simulink model "Guidance_Equations2"  (R2013a)
settings: Solver=ode4  StartTime=0.0  StopTime=10  FixedStep=0.01  RelTol=1e-3
undefined symbols (not defined in the file or in its folder): sigbuilder_block
settings Model: Creator=Ibrahim_B92  LastModifiedBy=Ibrahim_B92
settings DataIOCC: LimitDataPoints=off  SaveOutput=off

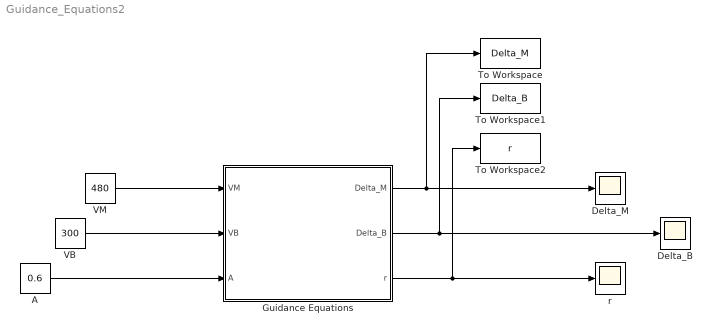
== system Guidance_Equations2 ==
  A : Constant  Value=0.6
  Delta_B : Scope
  Delta_M : Scope
      settings: YMin=0.6683  YMax=0.67
  Guidance Equations : Subsystem
  To Workspace : ToWorkspace  VariableName=Delta_M  SampleTime=-1
  To Workspace1 : ToWorkspace  VariableName=Delta_B  SampleTime=-1
  To Workspace2 : ToWorkspace  VariableName=r  SampleTime=-1
  VB : Constant  Value=300
  VM : Constant  Value=480
  r : Scope
      settings: SaveName=ScopeData2
  wires:
  VM/1 -> Guidance Equations/1(VM)
  VB/1 -> Guidance Equations/2(VB)
  Guidance Equations/1(Delta_M) -> Delta_M/1, To Workspace/1
  Guidance Equations/2(Delta_B) -> Delta_B/1, To Workspace1/1
  Guidance Equations/3(r) -> To Workspace2/1, r/1
  A/1 -> Guidance Equations/3(A)

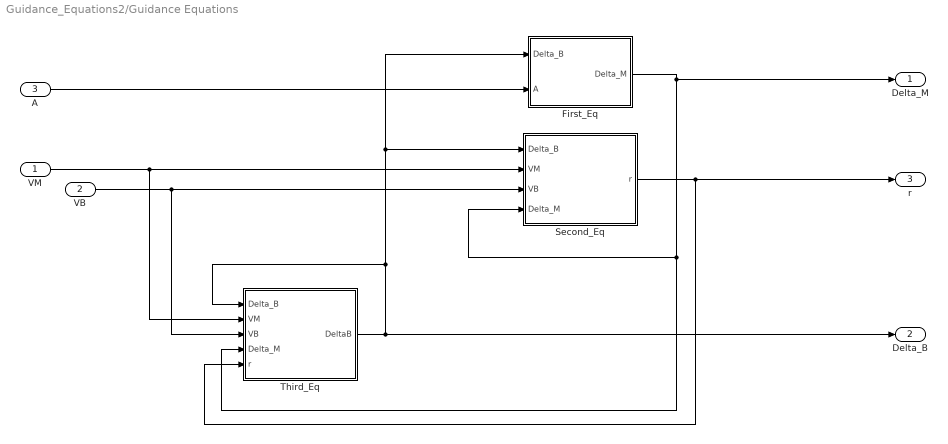
== system Guidance_Equations2/Guidance Equations ==
  VM : Inport
  VB : Inport  Port=2
  A : Inport  Port=3
  First_Eq : Subsystem
  Second_Eq : Subsystem
  Third_Eq : Subsystem
  Delta_M : Outport
  Delta_B : Outport  Port=2
  r : Outport  Port=3
  wires:
  Third_Eq/1(DeltaB) -> Second_Eq/1(Delta_B), First_Eq/1(Delta_B), Third_Eq/1(Delta_B), Delta_B/1
  First_Eq/1(Delta_M) -> Delta_M/1, Third_Eq/4(Delta_M), Second_Eq/4(Delta_M)
  VM/1 -> Third_Eq/2(VM), Second_Eq/2(VM)
  VB/1 -> Third_Eq/3(VB), Second_Eq/3(VB)
  Second_Eq/1(r) -> Third_Eq/5(r), r/1
  A/1 -> First_Eq/2(A)

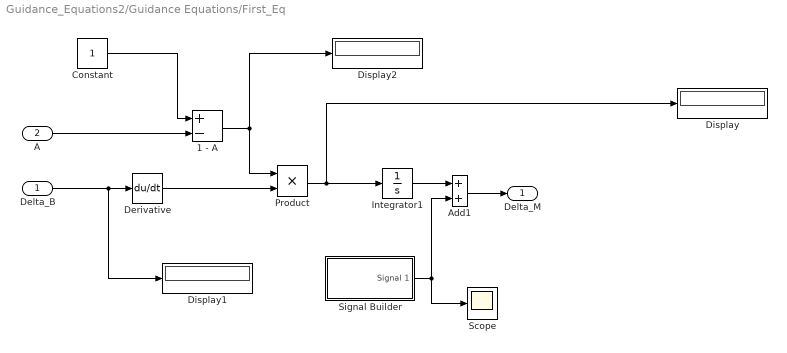
== system Guidance_Equations2/Guidance Equations/First_Eq ==
  Delta_B : Inport
  A : Inport  Port=2
  1 - A : Sum  Inputs=+-
  Add1 : Sum
  Constant : Constant
  Derivative : Derivative
  Display : Display
  Display1 : Display
  Display2 : Display
  Integrator1 : Integrator
  Product : Product
  Scope : Scope
      settings: SaveName=ScopeData4
  Signal Builder : Subsystem  Tag=STV Subsys  LoadFcn=sigbuilder_block('load',[437.25 118.5 550.5 394.5 ]);  StartFcn=sigbuilder_block('start');  StopFcn=sigbuilder_block('stop');  ClipboardFcn=sigbuilder_block('clipboard');  mask(Sigbuilder block){}
      mask help: Simulink:masks:SigbuilderBlock_MD
      mask init:
      | if ~strcmp(get_param(bdroot(gcbh),'SimulationStatus'),'stopped') tuvar = sigbuilder_block('maskInit'); end
      settings: CopyFcn=sigbuilder_block('copy');  DeleteFcn=sigbuilder_block('delete');  ModelCloseFcn=sigbuilder_block('modelClose');  PreSaveFcn=sigbuilder_block('preSave');  PauseFcn=sigbuilder_block('pause');  ContinueFcn=sigbuilder_block('continue');  NameChangeFcn=sigbuilder_block('namechange');  OpenFcn=sigbuilder_block('open',[437.25 118.5 550.5 394.5 ]);  CloseFcn=sigbuilder_block('close');
      mask Display: plot(0, 0, 100, 100,[2, 2, 32, 32, 2], [68, 8, 8, 68, 68],[32, 2], [38, 38], [32, 19, 2],[53, 60, 44], [32, 17, 17, 2],[16, 16, 31, 31]);txt = getActiveGroup(gcbh);text(2, 100, txt,'verticalAlignment', 'top');
  Delta_M : Outport
  wires:
  Delta_B/1 -> Display1/1, Derivative/1
  Derivative/1 -> Product/2
  Product/1 -> Display/1, Integrator1/1
  A/1 -> 1 - A/2
  Constant/1 -> 1 - A/1
  1 - A/1 -> Display2/1, Product/1
  Signal Builder/1(Signal 1) -> Add1/2, Scope/1
  Add1/1 -> Delta_M/1
  Integrator1/1 -> Add1/1

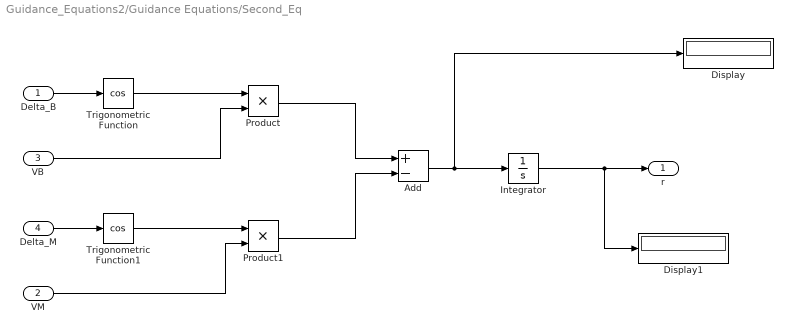
== system Guidance_Equations2/Guidance Equations/Second_Eq ==
  Delta_B : Inport
  VM : Inport  Port=2
  VB : Inport  Port=3
  Delta_M : Inport  Port=4
  Add : Sum  Inputs=+-
  Display : Display
  Display1 : Display
  Integrator : Integrator
  Product : Product
  Product1 : Product
  Trigonometric Function : Trigonometry  Operator=cos
  Trigonometric Function1 : Trigonometry  Operator=cos
  r : Outport
  wires:
  Delta_B/1 -> Trigonometric Function/1
  VB/1 -> Product/2
  VM/1 -> Product1/2
  Product/1 -> Add/1
  Product1/1 -> Add/2
  Add/1 -> Integrator/1, Display/1
  Delta_M/1 -> Trigonometric Function1/1
  Trigonometric Function1/1 -> Product1/1
  Trigonometric Function/1 -> Product/1
  Integrator/1 -> Display1/1, r/1

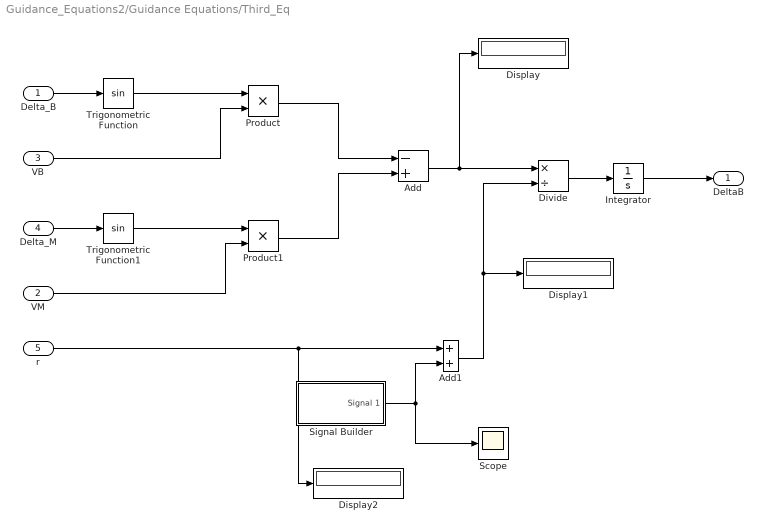
== system Guidance_Equations2/Guidance Equations/Third_Eq ==
  Delta_B : Inport
  VM : Inport  Port=2
  VB : Inport  Port=3
  Delta_M : Inport  Port=4
  r : Inport  Port=5
  Add : Sum  Inputs=-+
  Add1 : Sum
  Display : Display
  Display1 : Display
  Display2 : Display
  Divide : Product  Inputs=*/
  Integrator : Integrator
  Product : Product
  Product1 : Product
  Scope : Scope
      settings: SaveName=ScopeData3
  Signal Builder : Subsystem  Tag=STV Subsys  LoadFcn=sigbuilder_block('load');  StartFcn=sigbuilder_block('start');  StopFcn=sigbuilder_block('stop');  ClipboardFcn=sigbuilder_block('clipboard');  mask(Sigbuilder block){}
      mask help: Simulink:masks:SigbuilderBlock_MD
      mask init:
      | if ~strcmp(get_param(bdroot(gcbh),'SimulationStatus'),'stopped') tuvar = sigbuilder_block('maskInit'); end
      settings: CopyFcn=sigbuilder_block('copy');  DeleteFcn=sigbuilder_block('delete');  ModelCloseFcn=sigbuilder_block('modelClose');  PreSaveFcn=sigbuilder_block('preSave');  PauseFcn=sigbuilder_block('pause');  ContinueFcn=sigbuilder_block('continue');  NameChangeFcn=sigbuilder_block('namechange');  OpenFcn=sigbuilder_block('open',[437.25 118.5 550.5 394.5 ]);  CloseFcn=sigbuilder_block('close');
      mask Display: plot(0, 0, 100, 100,[2, 2, 32, 32, 2], [68, 8, 8, 68, 68],[32, 2], [38, 38], [32, 19, 2],[53, 60, 44], [32, 17, 17, 2],[16, 16, 31, 31]);txt = getActiveGroup(gcbh);text(2, 100, txt,'verticalAlignment', 'top');
  Trigonometric Function : Trigonometry
  Trigonometric Function1 : Trigonometry
  DeltaB : Outport
  wires:
  Delta_B/1 -> Trigonometric Function/1
  Delta_M/1 -> Trigonometric Function1/1
  VB/1 -> Product/2
  VM/1 -> Product1/2
  Integrator/1 -> DeltaB/1
  Add/1 -> Display/1, Divide/1
  Divide/1 -> Integrator/1
  r/1 -> Add1/1, Display2/1
  Trigonometric Function1/1 -> Product1/1
  Product/1 -> Add/1
  Product1/1 -> Add/2
  Trigonometric Function/1 -> Product/1
  Add1/1 -> Display1/1, Divide/2
  Signal Builder/1(Signal 1) -> Add1/2, Scope/1

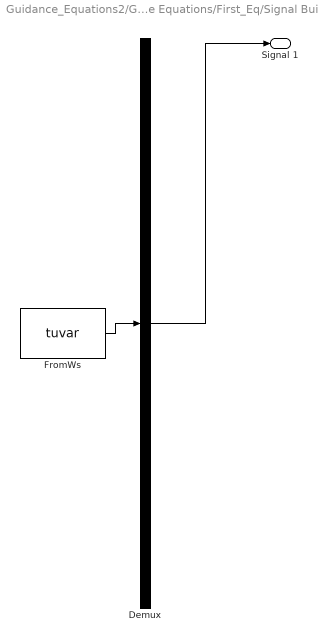
== system Guidance_Equations2/Guidance Equations/First_Eq/Signal Builder ==
  Demux : Demux  Tag=STV Demux  Outputs=1
  FromWs : FromWorkspace  Tag=STV FromWs  VariableName=tuvar  SampleTime=0
      SigBuilderData=|
      | common.afterFinalStr = 'Extrapolate'
      | common.sampleTime = 0
      | dataSet.timeRange = [0 10]
      | dataSet.name = 'Group 1'
      | sbobj.Groups.Name = 'Group 1'
      | sbobj.Groups.Signals.Name = 'Signal 1'
      | sbobj.Groups.Signals.XData = [0 0.01 0.01 10]
      | sbobj.Groups.Signals.YData = [1 1 0 0]
  Signal 1 : Outport  Tag=STV Outport
  wires:
  Demux/1 -> Signal 1/1
  FromWs/1 -> Demux/1

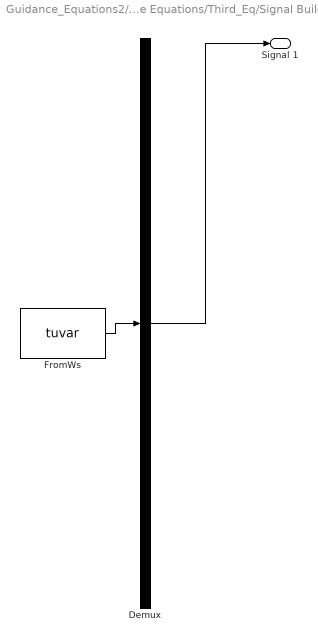
== system Guidance_Equations2/Guidance Equations/Third_Eq/Signal Builder ==
  Demux : Demux  Tag=STV Demux  Outputs=1
  FromWs : FromWorkspace  Tag=STV FromWs  VariableName=tuvar  SampleTime=0
      SigBuilderData=|
      | common.afterFinalStr = 'Extrapolate'
      | common.sampleTime = 0
      | dataSet.timeRange = [0 10]
      | dataSet.name = 'Group 1'
      | sbobj.Groups.Name = 'Group 1'
      | sbobj.Groups.Signals.Name = 'Signal 1'
      | sbobj.Groups.Signals.XData = [0 0.01 0.01 10]
      | sbobj.Groups.Signals.YData = [1 1 0 0]
  Signal 1 : Outport  Tag=STV Outport
  wires:
  Demux/1 -> Signal 1/1
  FromWs/1 -> Demux/1
